simulink subsystem "Kinematics"  (R2021a)
settings: Solver=VariableStepAuto  StartTime=0.0  StopTime=10.0  RelTol=1e-3
undefined symbols (not defined in the file): q0, r0
libraries: aerolibutil x1
settings Model: Creator=Laura  LastModifiedBy=Laura

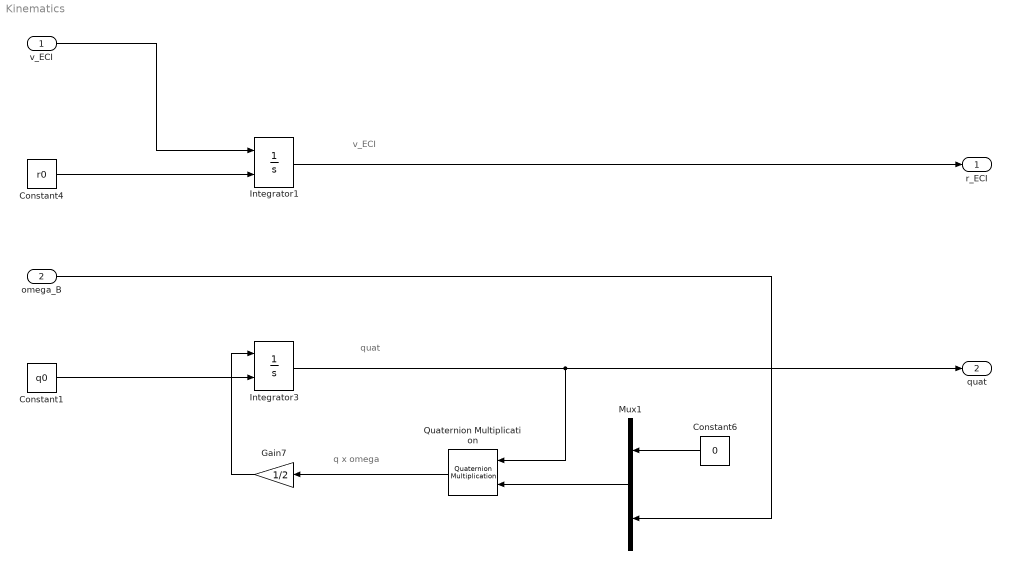
== system Kinematics ==
  note: q x omega
  note: quat
  note: v_ECI
  v_ECI : Inport
  omega_B : Inport  Port=2
  Constant1 : Constant  Value=q0
  Constant4 : Constant  Value=r0
  Constant6 : Constant  Value=0
  Gain7 : Gain  Gain=1/2
  Integrator1 : Integrator  InitialConditionSource=external
  Integrator3 : Integrator  InitialConditionSource=external
  Mux1 : Mux  Inputs=2
  Quaternion Multiplication : aerolibutil/Quaternion Multiplication
  r_ECI : Outport
  quat : Outport  Port=2
  wires:
  v_ECI/1 -> Integrator1/1
  Quaternion Multiplication/1 -> Gain7/1
  Constant1/1 -> Integrator3/2
  Constant6/1 -> Mux1/1
  Constant4/1 -> Integrator1/2
  Gain7/1 -> Integrator3/1
  Integrator1/1 -> r_ECI/1
  omega_B/1 -> Mux1/2
  Mux1/1 -> Quaternion Multiplication/2
  Integrator3/1 -> quat/1, Quaternion Multiplication/1
